simulink model "gap_generation_single_veh"  (R2019a)
settings: Solver=VariableStepAuto  StartTime=0.0  StopTime=35  FixedStep=0.1  MaxStep=0.05  RelTol=1e-3
libraries: simulink x21, powerlib_meascontrol x5, autolibshared x5
(part 3 of 3)

== stateflow chart gap_generation_single_veh/Fo/Chart ==
  state RegVehFoll
    during:
    u = regVehFollU;
  state AdjForLaneChange
    during:
    u = min(regVehFollU, virtualVehFollU);
  (default) -> RegVehFoll
  RegVehFoll -> AdjForLaneChange : [startAdjustment==1]
  data: regVehFollU input size=1; virtualVehFollU input size=1; startAdjustment input size=1; u output size=1

== stateflow chart gap_generation_single_veh/p1/Chart ==
  state RegVehFoll
    during:
    u = regVehFollU;
  state AdjForLaneChange
    during:
    u = min(regVehFollU, virtualVehFollU);
  (default) -> RegVehFoll
  RegVehFoll -> AdjForLaneChange : [startAdjustment==1]
  data: regVehFollU input size=1; virtualVehFollU input size=1; startAdjustment input size=1; u output size=1

== stateflow chart gap_generation_single_veh/Ld/Chart ==
  state RegVehFoll
    during:
    u = regVehFollU;
  state AdjForLaneChange
    during:
    u = min(regVehFollU, virtualVehFollU);
  (default) -> RegVehFoll
  RegVehFoll -> AdjForLaneChange : [startAdjustment==1]
  data: regVehFollU input size=1; virtualVehFollU input size=1; startAdjustment input size=1; u output size=1

== stateflow chart gap_generation_single_veh/Fd/Chart ==
  state RegVehFoll
    during:
    u = regVehFollU;
  state AdjForLaneChange
    during:
    u = min(regVehFollU, virtualVehFollU);
  (default) -> RegVehFoll
  RegVehFoll -> AdjForLaneChange : [startAdjustment==1]
  data: regVehFollU input size=1; virtualVehFollU input size=1; startAdjustment input size=1; u output size=1

== stateflow chart gap_generation_single_veh/Fd/Longitudinal Adjustments for Lane Change/Chart ==
  state VehFollowing
    during:
    u = uVehFoll;
    state = 0;
  state SpeedControl
    during:
    u = uVelControl;
    state = 1;
  (default) -> VehFollowing
  SpeedControl -> VehFollowing : [uVehFoll>=uVelControl]
  VehFollowing -> SpeedControl : [(velDiff>=0) && (uVehFoll<0)]
  data: state output size=1; u output size=1; velDiff input size=1; uVelControl input double; uVehFoll input size=1

== stateflow chart gap_generation_single_veh/Ld/Longitudinal Adjustments for Lane Change/Chart ==
  state VehFollowing
    during:
    u = uVehFoll;
    state = 0;
  state SpeedControl
    during:
    u = uVelControl;
    state = 1;
  (default) -> VehFollowing
  SpeedControl -> VehFollowing : [uVehFoll>=uVelControl]
  VehFollowing -> SpeedControl : [(velDiff>=0) && (uVehFoll<0)]
  data: state output size=1; u output size=1; velDiff input size=1; uVelControl input double; uVehFoll input size=1

== stateflow chart gap_generation_single_veh/Lo/Longitudinal Adjustments for Lane Change/Chart ==
  state VehFollowing
    during:
    u = uVehFoll;
    state = 0;
  state SpeedControl
    during:
    u = uVelControl;
    state = 1;
  (default) -> VehFollowing
  SpeedControl -> VehFollowing : [uVehFoll>=uVelControl]
  VehFollowing -> SpeedControl : [(velDiff>=0) && (uVehFoll<0)]
  data: state output size=1; u output size=1; velDiff input size=1; uVelControl input double; uVehFoll input size=1

== stateflow chart gap_generation_single_veh/p1/Longitudinal Adjustments for Lane Change/Chart ==
  state VehFollowing
    during:
    u = uVehFoll;
    state = 0;
  state SpeedControl
    during:
    u = uVelControl;
    state = 1;
  (default) -> VehFollowing
  SpeedControl -> VehFollowing : [uVehFoll>=uVelControl]
  VehFollowing -> SpeedControl : [(velDiff>=0) && (uVehFoll<0)]
  data: state output size=1; u output size=1; velDiff input size=1; uVelControl input double; uVehFoll input size=1

== stateflow chart gap_generation_single_veh/Fo/Longitudinal Adjustments for Lane Change/Chart ==
  state VehFollowing
    during:
    u = uVehFoll;
    state = 0;
  state SpeedControl
    during:
    u = uVelControl;
    state = 1;
  (default) -> VehFollowing
  SpeedControl -> VehFollowing : [uVehFoll>=uVelControl]
  VehFollowing -> SpeedControl : [(velDiff>=0) && (uVehFoll<0)]
  data: state output size=1; u output size=1; velDiff input size=1; uVelControl input double; uVehFoll input size=1
